simulink model "slave_task"  (Simulink 7.1)
libraries: mathlib x3, logiclib x2, inoutlib x1
settings Model: Creator=jsobota  LastModifiedBy=jsobota  ExtModeTrigMode=oneshot  ExtModeArmWhenConnect=off

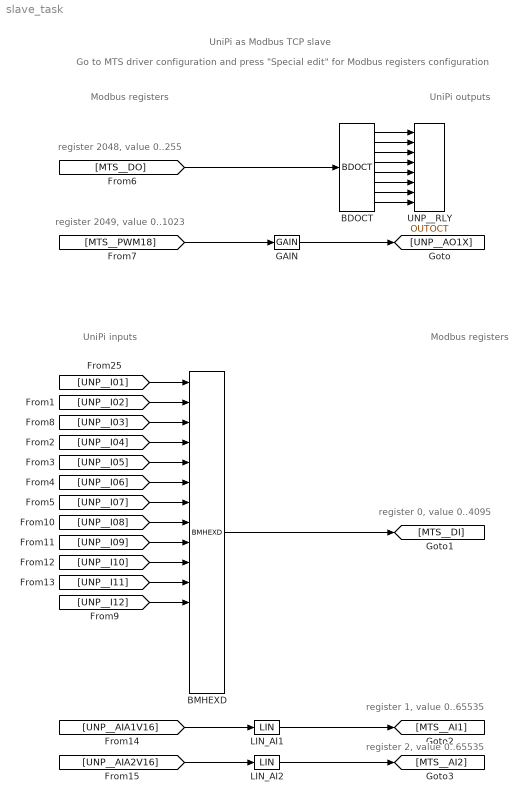
== system slave_task ==
  note: Modbus registers
  note: UniPi outputs
  note: UniPi inputs
  note: Modbus registers
  note: Go to MTS driver configuration and press "Special edit" for Modbus registers configuration
  note: UniPi as Modbus TCP slave
  note: register 2048, value 0..255
  note: register 2049, value 0..1023
  note: register 0, value 0..4095
  note: register 1, value 0..65535
  note: register 2, value 0..65535
  BDOCT : logiclib/BDOCT  shift=0
  BMHEXD : logiclib/BMHEXD  shift=0
  GAIN : mathlib/GAIN  k=1
  LIN_AI1 : mathlib/LIN  u1=0  y1=0  u2=10  y2=65535
  LIN_AI2 : mathlib/LIN  u1=0  y1=0  u2=10  y2=65535
  UNP__RLY : inoutlib/OUTOCT
  wires:
  BDOCT/1 -> UNP__RLY/1
  BDOCT/2 -> UNP__RLY/2
  BDOCT/3 -> UNP__RLY/3
  BDOCT/4 -> UNP__RLY/4
  BDOCT/5 -> UNP__RLY/5
  BDOCT/6 -> UNP__RLY/6
  BDOCT/7 -> UNP__RLY/7
  BDOCT/8 -> UNP__RLY/8
  BMHEXD/1 -> [MTS__DI]
  [UNP__I02] -> BMHEXD/2
  [UNP__I08] -> BMHEXD/8
  [UNP__I09] -> BMHEXD/9
  [UNP__I10] -> BMHEXD/10
  [UNP__I11] -> BMHEXD/11
  [UNP__AIA1V16] -> LIN_AI1/1
  [UNP__AIA2V16] -> LIN_AI2/1
  [UNP__I04] -> BMHEXD/4
  [UNP__I01] -> BMHEXD/1
  [UNP__I05] -> BMHEXD/5
  [UNP__I06] -> BMHEXD/6
  [UNP__I07] -> BMHEXD/7
  [MTS__DO] -> BDOCT/1
  [MTS__PWM18] -> GAIN/1
  [UNP__I03] -> BMHEXD/3
  [UNP__I12] -> BMHEXD/12
  GAIN/1 -> [UNP__AO1X]
  LIN_AI1/1 -> [MTS__AI1]
  LIN_AI2/1 -> [MTS__AI2]
